simulink model "model_with_phases"  (R2018b)
settings: Solver=daessc  StartTime=0.0  StopTime=1  RelTol=1e-3
StopFcn:
  | % fault = 10
  | %
  | %
  | %
  | %
  | % location = 160
  | %
  | %
  | %
  | %
  | %
  | %
  | % fault_data;
  | % simout=[simout,faults]
  | % simout(:,24) = location;
  | % data = xlsread('E:\testing data\test_data');
  | % data = [data;simout];
  | % xlswrite('E:\testing data\test_data',data);
libraries: powerlib x7, powerlib_meascontrol x2
settings Model: Creator=Edagotti Pavankumar  LastModifiedBy=Edagotti Pavankumar
settings SolverCC: ZeroCrossAlgorithm=Adaptive
settings DebuggingCC: IgnoredZcDiagnostic=none

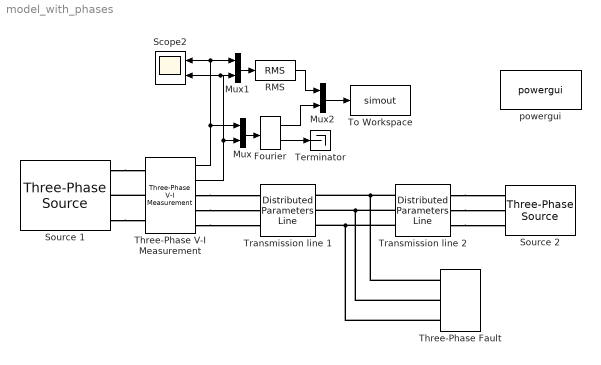
== system model_with_phases ==
  Fourier : powerlib_meascontrol/Measurements/Fourier  Freq=50  n=1  InInit=[0, 0]  Ts=0
      settings: SourceProductName=Simscape Power Systems
  Mux : Mux  Inputs=2
  Mux1 : Mux  Inputs=2
  Mux2 : Mux  Inputs=2
  RMS : powerlib_meascontrol/Measurements/RMS  TrueRMS=on  Freq=50  RMSInit=0  Ts=0
  Scope2 : Scope  NumInputPorts=2
  Source 1 : powerlib/Electrical Sources/Three-Phase Source  InternalConnection=Yg  VoltagePhases=off  Voltage=220e3  PhaseAngle=0  Voltage_phases=[25e3 25e3 25e3]/sqrt(3)  PhaseAngles_phases=[0 -120 +120]  Frequency=50  NonIdealSource=on  SpecifyImpedance=on  Resistance=0.8929  Inductance=16.58e-3  ShortCircuitLevel=100e6  BaseVoltage=220e3  XRratio=7  BusType=swing  Pref=10e3  Qref=0  Prefabc=[10e3, 10e3, 10e3]  Qrefabc=[0, 0, 0]  Qmin=-inf  Qmax=inf
  Source 2 : powerlib/Electrical Sources/Three-Phase Source  InternalConnection=Yg  VoltagePhases=off  Voltage=220e3  PhaseAngle=-40  Voltage_phases=[25e3 25e3 25e3]/sqrt(3)  PhaseAngles_phases=[0 -120 +120]  Frequency=50  NonIdealSource=on  SpecifyImpedance=on  Resistance=0.8929  Inductance=16.58e-3  ShortCircuitLevel=100e6  BaseVoltage=220e3  XRratio=7  BusType=PV  Pref=inf  Qref=0  Prefabc=[10e3, 10e3, 10e3]  Qrefabc=[0, 0, 0]  Qmin=-inf  Qmax=inf
  Terminator : Terminator
  Three-Phase V-I Measurement : powerlib/Measurements/Three-Phase V-I Measurement  VoltageMeasurement=phase-to-ground  SetLabelV=off  LabelV=Vabc  Vpu=on  VpuLL=off  CurrentMeasurement=yes  SetLabelI=off  LabelI=Iabc  Ipu=on  Pbase=100e6  Vbase=220e3  OutputType=Complex  PhasorSimulation=off  PSBequivalent=0
  Three-Phase Fault : powerlib/Elements/Three-Phase Fault  InitialStates=0  FaultA=on  FaultB=on  FaultC=on  GroundFault=off  SwitchTimes=0.5  External=off  SwitchStatus=NaN  FaultResistance=20  GroundResistance=0.001  SnubberResistance=1e6  SnubberCapacitance=inf  Measurements=None
  To Workspace : ToWorkspace  VariableName=simout  SampleTime=-1
      settings: MaxDataPoints=100  Save2DSignal=2-D array (concatenate along first dimension)
  Transmission line 1 : powerlib/Elements/Distributed Parameters Line  Phases=3  Frequency=50  Resistance=[0.0238 0.3885]  Inductance=[0.0009509508 0.0032508989]  Capacitance=[12.74e-9 7.751e-9]  Length=160  x1=[1.1933457766177e-09 256106.737010839 256106.737010841;314.159265358979 314.159265358979 314.159265358979;-0.264513808400128 -0.0183316743636763 -1.58912800115857]  x2=[1.31459963697142e-09 257720.72711148 257720.727111482;314.159265358979 314.159265358979 314.159265358979;-0.296611633434153 -0.0457482203169709 -1.61654454711186]  x3=[1.61711443767294e-12 793.390665840209 793.390665840219;314.159265358979 314.159265358979 314.159265358979;-0.74053676219142 -0.17619522013328 -1.74699154692818]  x4=[2.42615366680553e-12 1076.93135796091 1076.93135796092;314.159265358979 314.159265358979 314.159265358979;-0.1404290247802 -0.0783802254355058 -1.64917655223039]  x5=0.000803157247848664  V1=[1.193e-09 2.561e+05 2.561e+05;314.2 314.2 314.2;-0.2645 -0.01833 -1.589]  V2=[1.315e-09 2.577e+05 2.577e+05;314.2 314.2 314.2;-0.2966 -0.04575 -1.617]  I1=[1.617e-12 793.4 793.4;314.2 314.2 314.2;-0.7405 -0.1762 -1.747]  I2=[2.426e-12 1077 1077;314.2 314.2 314.2;-0.1404 -0.07838 -1.649]  nHarmo=1  Measurements=None
      settings: SourceProductName=Simscape Power Systems
  Transmission line 2 : powerlib/Elements/Distributed Parameters Line  Phases=3  Frequency=50  Resistance=[0.0238 0.3885]  Inductance=[0.0009509508 0.0032508989]  Capacitance=[12.74e-9 7.751e-9]  Length=40  x1=[1.31039976431671e-09 257720.72711148 257720.727111482;314.159265358979 314.159265358979 314.159265358979;-0.0964008186162161 0.08547021560208 -1.48532611119281]  x2=[1.27639148767729e-09 256920.332809657 256920.33280966;314.159265358979 314.159265358979 314.159265358979;-0.16586814746812 0.0790008961846271 -1.49179543061027]  x3=[1.45983024967746e-12 798.289373210209 798.289373210216;314.159265358979 314.159265358979 314.159265358979;2.31351999814091 0.129729677301775 -1.44106664949311]  x4=[2.33620147284963e-12 1084.26106264655 1084.26106264657;314.159265358979 314.159265358979 314.159265358979;0.179712254952421 0.00929096905672785 -1.56150535773818]  x5=0.000200789311962166  V1=[1.31e-09 2.577e+05 2.577e+05;314.2 314.2 314.2;-0.0964 0.08547 -1.485]  V2=[1.276e-09 2.569e+05 2.569e+05;314.2 314.2 314.2;-0.1659 0.079 -1.492]  I1=[1.46e-12 798.3 798.3;314.2 314.2 314.2;2.314 0.1297 -1.441]  I2=[2.336e-12 1084 1084;314.2 314.2 314.2;0.1797 0.009291 -1.562]  nHarmo=1  Measurements=None
      settings: SourceProductName=Simscape Power Systems
  powergui : powerlib/powergui  Priority=1  SimulationMode=Continuous  SampleTime=8.3333e-05  frequency=60  Iterations=50  frequencyindice=50  Pbase=100e6  ErrMax=1e-4  UnitsV=kV  UnitsW=MW  buscounter=0  FunctionMessages=off  echomessages=off  EnableUseOfTLC=off  CurrentSourceSwitches=off  DisableSnubberDevices=off  DisableRonSwitches=off  DisableVfSwitches=off  DisplayEquations=off  SolverType=Tustin/Backward Euler (TBE)  Interpol=off  ExternalGateDelay=off  methode=off  Ts=100  x0status=blocks  SPID=off  SwTol=0  HookPort=off  RestoreLinks=warning  ResistiveCurrentMeasurement=off  Frange=[0:2:500]  Ylog=off  Xlog=on  ShowGrid=off  save=off  variable=ZData  structure=0  ZoomFFT=off  StartTime=0.0  cycles=1  DisplayStyle=1  fundamental=60  FreqAxis=off  MaxFrequency=1000  frequencyindicesteady=1  RmsSteady=2  display=off
  wires:
  Fourier/1 -> Terminator/1
  Mux/1 -> Fourier/1
  Mux2/1 -> To Workspace/1
  Three-Phase V-I Measurement/2 -> Mux/2, Scope2/2, Mux1/2
  RMS/1 -> Mux2/1
  Three-Phase V-I Measurement/1 -> Mux/1, Mux1/1, Scope2/1
  Mux1/1 -> RMS/1
  Fourier/2 -> Mux2/2
  connections:
  Three-Phase V-I Measurement/RConn2 -- Transmission line 1/LConn2
  Three-Phase V-I Measurement/RConn1 -- Transmission line 1/LConn1
  Three-Phase V-I Measurement/RConn3 -- Transmission line 1/LConn3
  Source 1/RConn1 -- Three-Phase V-I Measurement/LConn1
  Transmission line 2/RConn1 -- Source 2/RConn1
  Transmission line 2/LConn2 -- Three-Phase Fault/LConn2 -- Transmission line 1/RConn2
  Transmission line 2/RConn2 -- Source 2/RConn2
  Source 1/RConn3 -- Three-Phase V-I Measurement/LConn3
  Transmission line 2/LConn3 -- Three-Phase Fault/LConn3 -- Transmission line 1/RConn3
  Three-Phase V-I Measurement/LConn2 -- Source 1/RConn2
  Transmission line 2/RConn3 -- Source 2/RConn3
  Transmission line 2/LConn1 -- Three-Phase Fault/LConn1 -- Transmission line 1/RConn1
